simulink model "ask_demod_channel"  (R2018a)
settings: Solver=VariableStepAuto  StartTime=0.0  StopTime=10.0  RelTol=1e-3
libraries: simulink x1, commrandsrc3 x1, commsynccomp2 x1
settings Model: Creator=hp  LastModifiedBy=hp

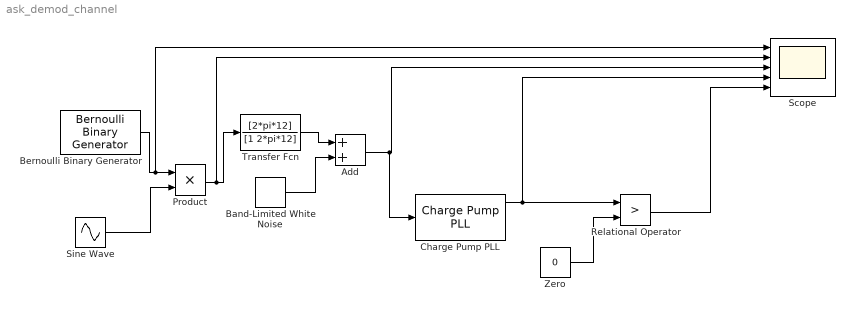
== system ask_demod_channel ==
  Add : Sum
  Band-Limited White Noise : simulink/Sources/Band-Limited White Noise  Cov=[0.0002]  Ts=0.1  seed=[23341]
  Bernoulli Binary Generator : commrandsrc3/Bernoulli Binary Generator  ProbabilityOfZero=0.3  SeedSource=Auto  Seed=0  SampleTime=1  SamplesPerFrame=1  OutputDataType=double  SimulateUsing=Interpreted execution
  Charge Pump PLL : commsynccomp2/Charge Pump PLL  Fn=[2*pi*1]  Fd=[1 2*pi*1]  Kvco=1  Fc=10  Ph=0  Ac=1
      settings: SourceProductName=Communications System Toolbox  SourceProductBaseCode=CM
  Product : Product
  Relational Operator : RelationalOperator  Operator=>  OutDataTypeStr=boolean  RndMeth=Simplest
  Scope : Scope  NumInputPorts=5
  Sine Wave : Sin  Frequency=2*pi*12  Samples=0.02  SampleTime=0.01
  Transfer Fcn : TransferFcn  Numerator=[2*pi*12]  Denominator=[1 2*pi*12]
  Zero : Constant  Value=0
  wires:
  Bernoulli Binary Generator/1 -> Product/1, Scope/1
  Sine Wave/1 -> Product/2
  Transfer Fcn/1 -> Add/1
  Band-Limited White Noise/1 -> Add/2
  Add/1 -> Charge Pump PLL/1, Scope/3
  Charge Pump PLL/1 -> Relational Operator/1, Scope/4
  Zero/1 -> Relational Operator/2
  Relational Operator/1 -> Scope/5
  Product/1 -> Scope/2, Transfer Fcn/1
